simulink model "compare"  (R2018b)
settings: Solver=ode45  StartTime=0.0  StopTime=100  RelTol=1e-3
libraries: neural x79
(part 1 of 4)
settings Model: Creator=abinwa  LastModifiedBy=abinwa

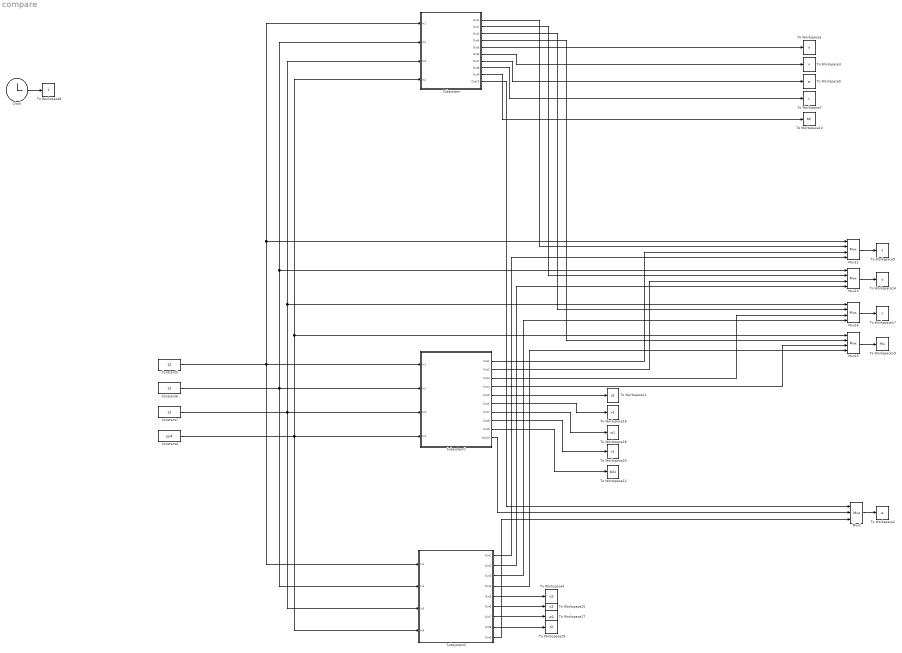
== system compare ==
  Clock : Clock
  Constant4 : Constant  Value=pi/4
  Constant5 : Constant  Value=12
  Constant6 : Constant  Value=12
  Constant7 : Constant  Value=12
  Mux1 : Mux  Inputs=3
  Mux{12..15} (4 alike) : Mux
  Subsystem : Subsystem
  Subsystem1 : Subsystem
  Subsystem2 : Subsystem
  To Workspace1 : ToWorkspace  VariableName=u  SampleTime=-1
  To Workspace10 : ToWorkspace  VariableName=tol  SampleTime=-1
  To Workspace11 : ToWorkspace  VariableName=u1  SampleTime=-1
  To Workspace12 : ToWorkspace  VariableName=tol1  SampleTime=-1
  To Workspace14 : ToWorkspace  VariableName=y  SampleTime=-1
  To Workspace16 : ToWorkspace  VariableName=v1  SampleTime=-1
  To Workspace17 : ToWorkspace  VariableName=z  SampleTime=-1
  To Workspace18 : ToWorkspace  VariableName=w1  SampleTime=-1
  To Workspace19 : ToWorkspace  VariableName=Psi  SampleTime=-1
  To Workspace2 : ToWorkspace  VariableName=e  SampleTime=-1
  To Workspace20 : ToWorkspace  VariableName=r1  SampleTime=-1
  To Workspace25 : ToWorkspace  VariableName=v2  SampleTime=-1
  To Workspace27 : ToWorkspace  VariableName=w2  SampleTime=-1
  To Workspace29 : ToWorkspace  VariableName=r2  SampleTime=-1
  To Workspace3 : ToWorkspace  VariableName=v  SampleTime=-1
  To Workspace4 : ToWorkspace  VariableName=u2  SampleTime=-1
  To Workspace5 : ToWorkspace  VariableName=w  SampleTime=-1
  To Workspace7 : ToWorkspace  VariableName=r  SampleTime=-1
  To Workspace8 : ToWorkspace  VariableName=t  SampleTime=-1
  To Workspace9 : ToWorkspace  VariableName=x  SampleTime=-1
  wires:
  Clock/1 -> To Workspace8/1
  Subsystem/1(Out1) -> Mux12/2
  Subsystem/2(Out2) -> Mux13/2
  Subsystem/3(Out3) -> Mux14/2
  Subsystem/4(Out4) -> Mux15/2
  Subsystem/5(Out5) -> To Workspace1/1
  Subsystem/6(Out6) -> To Workspace3/1
  Subsystem/7(Out7) -> To Workspace5/1
  Subsystem/8(Out8) -> To Workspace7/1
  Subsystem/9(Out9) -> To Workspace10/1
  Subsystem/10(Out10) -> Mux1/1
  Mux12/1 -> To Workspace9/1
  Mux13/1 -> To Workspace14/1
  Mux15/1 -> To Workspace19/1
  Constant5/1 -> Subsystem2/1(In1), Subsystem/1(In1), Mux12/1, Subsystem1/1(In1)
  Mux14/1 -> To Workspace17/1
  Constant6/1 -> Subsystem2/2(In2), Subsystem/2(In2), Mux13/1, Subsystem1/2(In2)
  Constant7/1 -> Subsystem2/3(In3), Subsystem1/3(In3), Subsystem/3(In3), Mux14/1
  Constant4/1 -> Subsystem2/4(In4), Subsystem1/4(In4), Subsystem/4(In4), Mux15/1
  Subsystem1/1(Out1) -> Mux12/3
  Subsystem1/2(Out2) -> Mux13/3
  Subsystem1/3(Out3) -> Mux14/3
  Subsystem1/4(Out4) -> Mux15/3
  Subsystem1/5(Out5) -> To Workspace11/1
  Subsystem1/6(Out6) -> To Workspace16/1
  Subsystem1/7(Out7) -> To Workspace18/1
  Subsystem1/8(Out8) -> To Workspace20/1
  Subsystem1/9(Out9) -> To Workspace12/1
  Subsystem1/10(Out10) -> Mux1/2
  Mux1/1 -> To Workspace2/1
  Subsystem2/1(Out1) -> Mux12/4
  Subsystem2/2(Out2) -> Mux13/4
  Subsystem2/3(Out3) -> Mux14/4
  Subsystem2/4(Out4) -> Mux15/4
  Subsystem2/5(Out5) -> To Workspace4/1
  Subsystem2/6(Out6) -> To Workspace25/1
  Subsystem2/7(Out7) -> To Workspace27/1
  Subsystem2/8(Out8) -> To Workspace29/1
  Subsystem2/9(Out9) -> Mux1/3

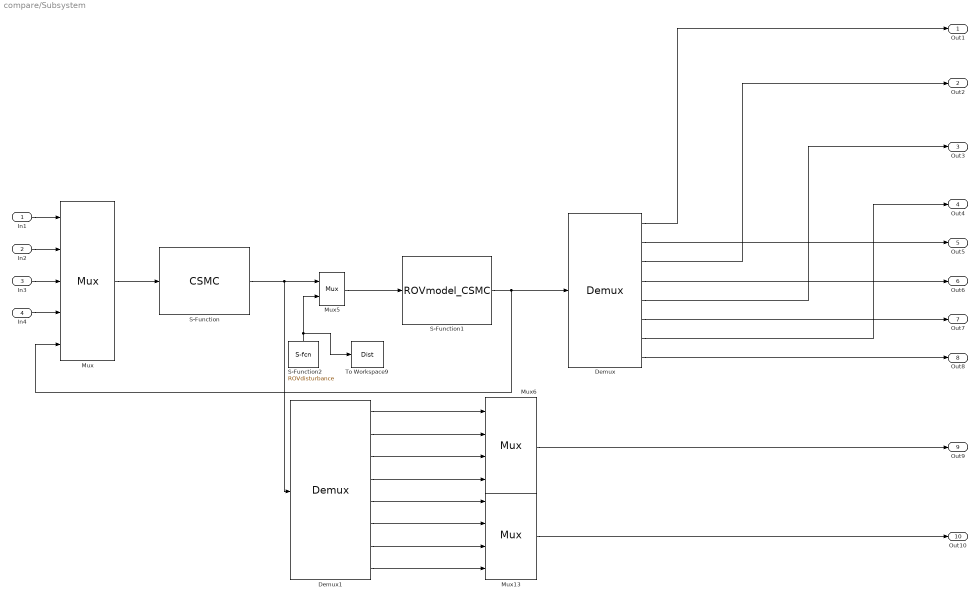
== system compare/Subsystem ==
  In1 : Inport
  In2 : Inport  Port=2
  In3 : Inport  Port=3
  In4 : Inport  Port=4
  Demux : Demux  Outputs=8
  Demux1 : Demux  Outputs=8
  Mux : Mux  Inputs=5
  Mux13 : Mux
  Mux5 : Mux  Inputs=2
  Mux6 : Mux
  S-Function : S-Function  FunctionName=CSMC  SFunctionDeploymentMode=off  EnableBusSupport=off
  S-Function1 : S-Function  FunctionName=ROVmodel_CSMC  SFunctionDeploymentMode=off  EnableBusSupport=off
  S-Function2 : S-Function  FunctionName=ROVdisturbance  SFunctionDeploymentMode=off  EnableBusSupport=off
  To Workspace9 : ToWorkspace  VariableName=Dist  SampleTime=-1
  Out1 : Outport
  Out2 : Outport  Port=2
  Out3 : Outport  Port=3
  Out4 : Outport  Port=4
  Out5 : Outport  Port=5
  Out6 : Outport  Port=6
  Out7 : Outport  Port=7
  Out8 : Outport  Port=8
  Out9 : Outport  Port=9
  Out10 : Outport  Port=10
  wires:
  Demux1/4 -> Mux6/4
  S-Function1/1 -> Demux/1, Mux/5
  Demux1/5 -> Mux13/1
  Demux/8 -> Out8/1
  Demux/5 -> Out3/1
  In3/1 -> Mux/3
  Demux1/1 -> Mux6/1
  Demux1/3 -> Mux6/3
  Demux1/2 -> Mux6/2
  Demux/7 -> Out4/1
  Mux5/1 -> S-Function1/1
  S-Function/1 -> Mux5/1, Demux1/1
  S-Function2/1 -> Mux5/2, To Workspace9/1
  Mux/1 -> S-Function/1
  Demux1/7 -> Mux13/3
  Demux1/6 -> Mux13/2
  Mux13/1 -> Out10/1
  Demux1/8 -> Mux13/4
  In1/1 -> Mux/1
  Demux/4 -> Out6/1
  In2/1 -> Mux/2
  Mux6/1 -> Out9/1
  Demux/3 -> Out2/1
  Demux/6 -> Out7/1
  Demux/2 -> Out5/1
  In4/1 -> Mux/4
  Demux/1 -> Out1/1

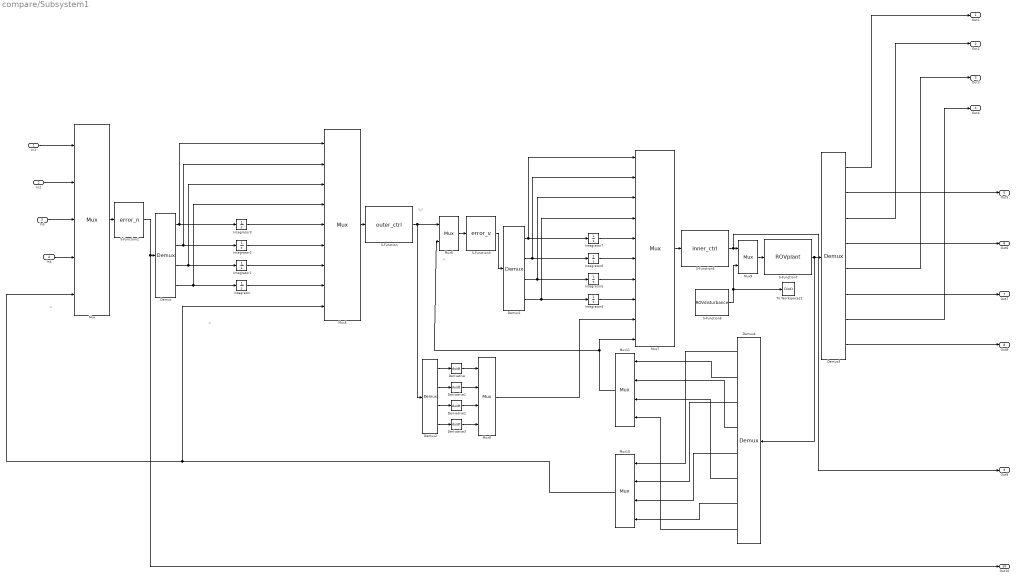
== system compare/Subsystem1 ==
  note: v_r
  note: n
  note: v
  note: n
  In1 : Inport
  In2 : Inport  Port=2
  In3 : Inport  Port=3
  In4 : Inport  Port=4
  Demux : Demux
  Demux1 : Demux
  Demux2 : Demux
  Demux3 : Demux  Outputs=8
  Demux4 : Demux  Outputs=8
  Derivative{,1..3} (4 alike) : Derivative
  Integrator{,1..7} (8 alike) : Integrator
  Mux : Mux  Inputs=5
  Mux10 : Mux
  Mux11 : Mux
  Mux5 : Mux  Inputs=9
  Mux6 : Mux  Inputs=2
  Mux7 : Mux  Inputs=10
  Mux8 : Mux
  Mux9 : Mux  Inputs=2
  S-Function : S-Function  FunctionName=outer_ctrl  SFunctionDeploymentMode=off  EnableBusSupport=off
  S-Function2 : S-Function  FunctionName=error_n  SFunctionDeploymentMode=off  EnableBusSupport=off
  S-Function3 : S-Function  FunctionName=error_v  SFunctionDeploymentMode=off  EnableBusSupport=off
  S-Function5 : S-Function  FunctionName=inner_ctrl  SFunctionDeploymentMode=off  EnableBusSupport=off
  S-Function6 : S-Function  FunctionName=ROVdisturbance  SFunctionDeploymentMode=off  EnableBusSupport=off
  S-Function7 : S-Function  FunctionName=ROVplant  SFunctionDeploymentMode=off  EnableBusSupport=off
  To Workspace21 : ToWorkspace  VariableName=Dist1  SampleTime=-1
  Out1 : Outport
  Out2 : Outport  Port=2
  Out3 : Outport  Port=3
  Out4 : Outport  Port=4
  Out5 : Outport  Port=5
  Out6 : Outport  Port=6
  Out7 : Outport  Port=7
  Out8 : Outport  Port=8
  Out9 : Outport  Port=9
  Out10 : Outport  Port=10
  wires:
  Demux1/4 -> Mux7/4, Integrator4/1
  S-Function6/1 -> To Workspace21/1, Mux9/2
  Mux8/1 -> Mux7/9
  Demux1/3 -> Mux7/3, Integrator5/1
  Demux2/2 -> Derivative1/1
  Demux4/5 -> Mux10/3
  Integrator/1 -> Mux5/8
  S-Function/1 -> Demux2/1, Mux6/1
  Integrator6/1 -> Mux7/6
  Integrator7/1 -> Mux7/5
  Mux9/1 -> S-Function7/1
  Mux10/1 -> Mux5/9, Mux/5
  Derivative3/1 -> Mux8/4
  Demux/1 -> Integrator3/1, Mux5/1
  Derivative2/1 -> Mux8/3
  S-Function3/1 -> Demux1/1
  S-Function7/1 -> Demux4/1, Demux3/1
  S-Function2/1 -> Out10/1, Demux/1
  Derivative/1 -> Mux8/1
  Demux4/2 -> Mux11/1
  Demux1/1 -> Mux7/1, Integrator7/1
  Mux11/1 -> Mux7/10, Mux6/2
  Mux5/1 -> S-Function/1
  Demux3/7 -> Out4/1
  Demux/4 -> Integrator/1, Mux5/4
  Demux2/3 -> Derivative2/1
  Integrator4/1 -> Mux7/8
  Mux/1 -> S-Function2/1
  Integrator2/1 -> Mux5/6
  Demux/2 -> Integrator2/1, Mux5/2
  Demux/3 -> Integrator1/1, Mux5/3
  Demux4/3 -> Mux10/2
  Derivative1/1 -> Mux8/2
  Mux6/1 -> S-Function3/1
  Demux3/1 -> Out1/1
  Mux7/1 -> S-Function5/1
  Integrator3/1 -> Mux5/5
  Demux4/4 -> Mux11/2
  Demux3/3 -> Out2/1
  Integrator1/1 -> Mux5/7
  Demux3/2 -> Out5/1
  Demux4/6 -> Mux11/3
  Integrator5/1 -> Mux7/7
  Demux4/8 -> Mux11/4
  Demux3/8 -> Out8/1
  Demux2/4 -> Derivative3/1
  Demux2/1 -> Derivative/1
  S-Function5/1 -> Out9/1, Mux9/1
  Demux1/2 -> Mux7/2, Integrator6/1
  Demux4/7 -> Mux10/4
  Demux4/1 -> Mux10/1
  In3/1 -> Mux/3
  Demux3/4 -> Out6/1
  In4/1 -> Mux/4
  Demux3/5 -> Out3/1
  Demux3/6 -> Out7/1
  In2/1 -> Mux/2
  In1/1 -> Mux/1

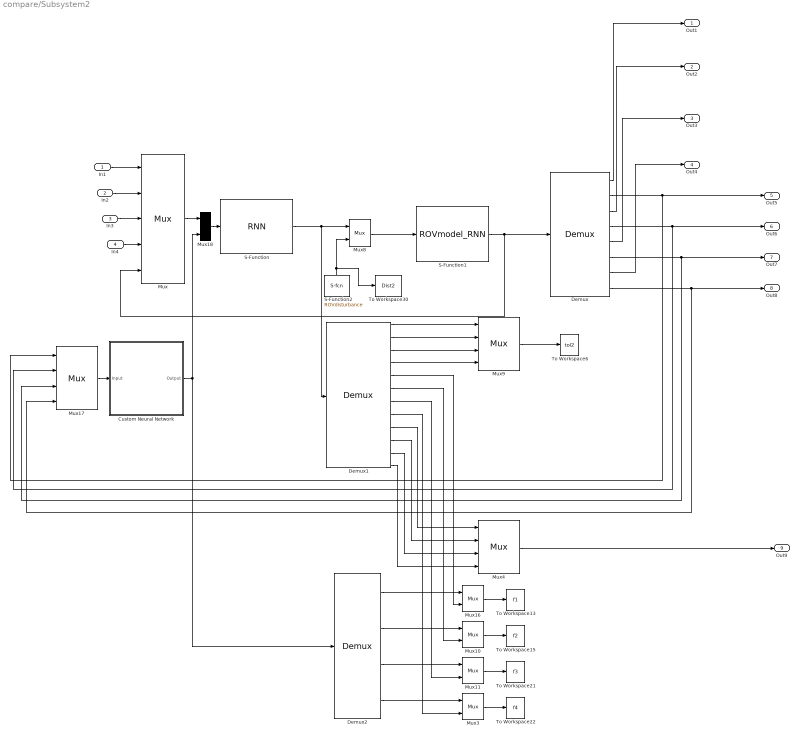
== system compare/Subsystem2 ==
  In1 : Inport
  In2 : Inport  Port=2
  In3 : Inport  Port=3
  In4 : Inport  Port=4
  Custom Neural Network : Subsystem  mask{ai_layer_1_delayed_1=[0;0;0;0;0;0;0;0;0;0;0;0;0;0;0;0;0;0;0;0], ai_layer_2_delayed_1=[0;0;0;0;0;0;0;0;0;0;0;0;0;0;0]}
      mask prompts: ai_layer_1_delayed_1 "Initial layer 1 state at timestep 0."; ai_layer_2_delayed_1 "Initial layer 2 state at timestep 0."
      mask help: Custom Neural Network
      mask Display: e = 0.06;c1 = [120 150 230]/255;c2 = ([120 150 230]+0)/383;c3 = ([120 150 230]+128)/383;patch([0 1 1 0],[0 0 1 1],c1);patch([0 1 1 1-e 1-e 0+e],[0 0 1 1-e 0+e 0+e],c2);patch([0 0 1 1-e 0+e 0+e],[0 1 1 1-e 1-e 0+e],c3);plot([0 1 1 0 0],[0 0 1 1 0]);fprintf('NNET');port_label('input',1,' Input');port_label('output',1,'Output ');
  Demux : Demux  Outputs=8
  Demux1 : Demux  Outputs=12
  Demux2 : Demux
  Mux : Mux  Inputs=5
  Mux{3,8,10..11,16,18} (6 alike) : Mux  Inputs=2
  Mux17 : Mux
  Mux4 : Mux
  Mux9 : Mux
  S-Function : S-Function  FunctionName=RNN  SFunctionDeploymentMode=off  EnableBusSupport=off
  S-Function1 : S-Function  FunctionName=ROVmodel_RNN  SFunctionDeploymentMode=off  EnableBusSupport=off
  S-Function2 : S-Function  FunctionName=ROVdisturbance  SFunctionDeploymentMode=off  EnableBusSupport=off
  To Workspace13 : ToWorkspace  VariableName=f1  SampleTime=-1
  To Workspace15 : ToWorkspace  VariableName=f2  SampleTime=-1
  To Workspace21 : ToWorkspace  VariableName=f3  SampleTime=-1
  To Workspace22 : ToWorkspace  VariableName=f4  SampleTime=-1
  To Workspace30 : ToWorkspace  VariableName=Dist2  SampleTime=-1
  To Workspace6 : ToWorkspace  VariableName=tol2  SampleTime=-1
  Out1 : Outport
  Out2 : Outport  Port=2
  Out3 : Outport  Port=3
  Out4 : Outport  Port=4
  Out5 : Outport  Port=5
  Out6 : Outport  Port=6
  Out7 : Outport  Port=7
  Out8 : Outport  Port=8
  Out9 : Outport  Port=9
  wires:
  Demux2/3 -> Mux11/1
  S-Function1/1 -> Demux/1, Mux/5
  Demux/4 -> Out6/1, Mux17/2
  Demux/2 -> Out5/1, Mux17/1
  Demux1/10 -> Mux4/2
  Demux2/2 -> Mux10/1
  Mux11/1 -> To Workspace21/1
  Demux1/6 -> Mux10/2
  In3/1 -> Mux/3
  In1/1 -> Mux/1
  Demux1/1 -> Mux9/1
  Demux/6 -> Out7/1, Mux17/3
  Demux1/4 -> Mux9/4
  Demux1/12 -> Mux4/4
  Mux9/1 -> To Workspace6/1
  Demux1/2 -> Mux9/2
  Mux18/1 -> S-Function/1
  Mux8/1 -> S-Function1/1
  Mux17/1 -> Custom Neural Network/1(Input)
  Demux1/5 -> Mux16/2
  S-Function/1 -> Mux8/1, Demux1/1
  Custom Neural Network/1(Output) -> Mux18/2, Demux2/1
  Demux/3 -> Out2/1
  Demux2/4 -> Mux3/1
  Mux3/1 -> To Workspace22/1
  Mux16/1 -> To Workspace13/1
  Demux/5 -> Out3/1
  Demux1/9 -> Mux4/1
  In2/1 -> Mux/2
  Demux1/11 -> Mux4/3
  Demux/8 -> Out8/1, Mux17/4
  Demux1/8 -> Mux3/2
  Mux/1 -> Mux18/1
  S-Function2/1 -> Mux8/2, To Workspace30/1
  Demux1/7 -> Mux11/2
  Demux2/1 -> Mux16/1
  Mux10/1 -> To Workspace15/1
  Demux1/3 -> Mux9/3
  Demux/7 -> Out4/1
  In4/1 -> Mux/4
  Demux/1 -> Out1/1
  Mux4/1 -> Out9/1

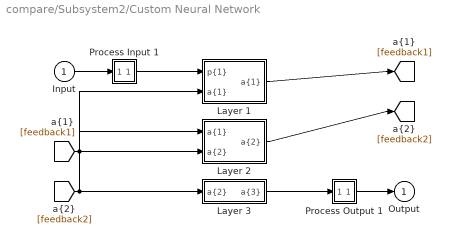
== system compare/Subsystem2/Custom Neural Network ==
  Input : Inport  PortDimensions=4  SampleTime=1
      mask Display: e = 0.06;c1 = [120 230 180]/255;c2 = ([120 230 180]+0)/(256+128);c3 = ([120 230 180]+128)/(256+128);patch([0 1 1 0],[0 0 1 1],c1);patch([0 1 1 1-e 1-e 0+e],[0 0 1 1-e 0+e 0+e],c2);patch([0 0 1 1-e 0+e 0+e],[0 1 1 1-e 1-e 0+e],c3);plot([0 1 1 0 0],[0 0 1 1 0]);
  Layer 1 : Subsystem
      mask Display: e = 0.06;c1 = [120 150 230]/255;c2 = ([120 150 230]+0)/383;c3 = ([120 150 230]+128)/383;patch([0 1 1 0],[0 0 1 1],c1);patch([0 1 1 1-e 1-e 0+e],[0 0 1 1-e 0+e 0+e],c2);patch([0 0 1 1-e 0+e 0+e],[0 1 1 1-e 1-e 0+e],c3);plot([0 1 1 0 0],[0 0 1 1 0]);
  Layer 2 : Subsystem
      mask Display: e = 0.06;c1 = [120 150 230]/255;c2 = ([120 150 230]+0)/383;c3 = ([120 150 230]+128)/383;patch([0 1 1 0],[0 0 1 1],c1);patch([0 1 1 1-e 1-e 0+e],[0 0 1 1-e 0+e 0+e],c2);patch([0 0 1 1-e 0+e 0+e],[0 1 1 1-e 1-e 0+e],c3);plot([0 1 1 0 0],[0 0 1 1 0]);
  Layer 3 : Subsystem
      mask Display: e = 0.06;c1 = [120 150 230]/255;c2 = ([120 150 230]+0)/383;c3 = ([120 150 230]+128)/383;patch([0 1 1 0],[0 0 1 1],c1);patch([0 1 1 1-e 1-e 0+e],[0 0 1 1-e 0+e 0+e],c2);patch([0 0 1 1-e 0+e 0+e],[0 1 1 1-e 1-e 0+e],c3);plot([0 1 1 0 0],[0 0 1 1 0]);
  Process Input 1 : Subsystem
      mask Display: e = 0.06;c1 = [120 150 230]/255;c2 = ([120 150 230]+0)/383;c3 = ([120 150 230]+128)/383;patch([0 1 1 0],[0 0 1 1],c1);patch([0 1 1 1-e 1-e 0+e],[0 0 1 1-e 0+e 0+e],c2);patch([0 0 1 1-e 0+e 0+e],[0 1 1 1-e 1-e 0+e],c3);plot([0 1 1 0 0],[0 0 1 1 0]);
  Process Output 1 : Subsystem
      mask Display: e = 0.06;c1 = [120 150 230]/255;c2 = ([120 150 230]+0)/383;c3 = ([120 150 230]+128)/383;patch([0 1 1 0],[0 0 1 1],c1);patch([0 1 1 1-e 1-e 0+e],[0 0 1 1-e 0+e 0+e],c2);patch([0 0 1 1-e 0+e 0+e],[0 1 1 1-e 1-e 0+e],c3);plot([0 1 1 0 0],[0 0 1 1 0]);
  Output : Outport  InitialOutput=[0;0;0;0]
      mask Display: e = 0.06;c1 = [120 230 180]/255;c2 = ([120 230 180]+0)/(256+128);c3 = ([120 230 180]+128)/(256+128);patch([0 1 1 0],[0 0 1 1],c1);patch([0 1 1 1-e 1-e 0+e],[0 0 1 1-e 0+e 0+e],c2);patch([0 0 1 1-e 0+e 0+e],[0 1 1 1-e 1-e 0+e],c3);plot([0 1 1 0 0],[0 0 1 1 0]);
  wires:
  Input/1 -> Process Input 1/1(x)
  Process Output 1/1(y) -> Output/1
  Process Input 1/1(p) -> Layer 1/1("p{1}")
  Layer 1/1("a{1}") -> [feedback1]
  [feedback1] -> Layer 1/2("a{1} "), Layer 2/1("a{1} ")
  Layer 2/1("a{2}") -> [feedback2]
  [feedback2] -> Layer 2/2("a{2} "), Layer 3/1("a{2} ")
  Layer 3/1("a{3}") -> Process Output 1/1(a)

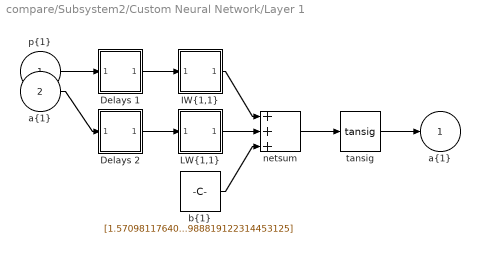
== system compare/Subsystem2/Custom Neural Network/Layer 1 ==
  "p{1}" : Inport  PortDimensions=4  SampleTime=1
      mask Display: e = 0.06;c1 = [120 230 180]/255;c2 = ([120 230 180]+0)/(256+128);c3 = ([120 230 180]+128)/(256+128);patch([0 1 1 0],[0 0 1 1],c1);patch([0 1 1 1-e 1-e 0+e],[0 0 1 1-e 0+e 0+e],c2);patch([0 0 1 1-e 0+e 0+e],[0 1 1 1-e 1-e 0+e],c3);plot([0 1 1 0 0],[0 0 1 1 0]);
  "a{1} " : Inport  Port=2  PortDimensions=20  SampleTime=1
      mask Display: e = 0.06;c1 = [120 230 180]/255;c2 = ([120 230 180]+0)/(256+128);c3 = ([120 230 180]+128)/(256+128);patch([0 1 1 0],[0 0 1 1],c1);patch([0 1 1 1-e 1-e 0+e],[0 0 1 1-e 0+e 0+e],c2);patch([0 0 1 1-e 0+e 0+e],[0 1 1 1-e 1-e 0+e],c3);plot([0 1 1 0 0],[0 0 1 1 0]);
  Delays 1 : Subsystem
      mask Display: e = 0.06;c1 = [120 150 230]/255;c2 = ([120 150 230]+0)/383;c3 = ([120 150 230]+128)/383;patch([0 1 1 0],[0 0 1 1],c1);patch([0 1 1 1-e 1-e 0+e],[0 0 1 1-e 0+e 0+e],c2);patch([0 0 1 1-e 0+e 0+e],[0 1 1 1-e 1-e 0+e],c3);plot([0 1 1 0 0],[0 0 1 1 0]);disp('0');
  Delays 2 : Subsystem
      mask Display: e = 0.06;c1 = [120 150 230]/255;c2 = ([120 150 230]+0)/383;c3 = ([120 150 230]+128)/383;patch([0 1 1 0],[0 0 1 1],c1);patch([0 1 1 1-e 1-e 0+e],[0 0 1 1-e 0+e 0+e],c2);patch([0 0 1 1-e 0+e 0+e],[0 1 1 1-e 1-e 0+e],c3);plot([0 1 1 0 0],[0 0 1 1 0]);disp('1');
  "IW{1,1}" : Subsystem
      mask Display: e = 0.06;c1 = [120 150 230]/255;c2 = ([120 150 230]+0)/383;c3 = ([120 150 230]+128)/383;patch([0 1 1 0],[0 0 1 1],c1);patch([0 1 1 1-e 1-e 0+e],[0 0 1 1-e 0+e 0+e],c2);patch([0 0 1 1-e 0+e 0+e],[0 1 1 1-e 1-e 0+e],c3);plot([0 1 1 0 0],[0 0 1 1 0]);disp('W');
  "LW{1,1}" : Subsystem
      mask Display: e = 0.06;c1 = [120 150 230]/255;c2 = ([120 150 230]+0)/383;c3 = ([120 150 230]+128)/383;patch([0 1 1 0],[0 0 1 1],c1);patch([0 1 1 1-e 1-e 0+e],[0 0 1 1-e 0+e 0+e],c2);patch([0 0 1 1-e 0+e 0+e],[0 1 1 1-e 1-e 0+e],c3);plot([0 1 1 0 0],[0 0 1 1 0]);disp('W');
  "b{1}" : Constant  Value=[1.5709811764087333596506823596428148448467254638671875;-1.422432849296332957322874790406785905361175537109375;1.257830636243737476576143308193422853946685791015625;-1.0965606272778114504973245857399888336658477783203125;-0.93559678076312768890687721068388782441616058349609375;-0.73655566333232591613722206602687947452068328857421875;-0.50859059257384853225403276155702769756317138671875;-0.3661309918072708224912048535770736634731292724609375;0.2362124825473512768070349920890294015407562255859375;0.0871527292053556890127907763599068857729434967041015625;-0.09220173179144837416476576663626474328339099884033203125;0.201297008489096651562277884295326657593250274658203125;0.40818274931037457076143937229062430560588836669921875;-0.612669858552886470448584077530540525913238525390625;0.79439985267361856724477320312871597707271575927734375;0.8775296810612600584278197857202030718326568603515625;1.0930187382606926238537425888353027403354644775390625;1.2798307915173892101989849834353663027286529541015625;-1.3805805253881249239356066027539782226085662841796875;-1.5889086928901339224040611952659673988819122314453125]
      mask Display: e = 0.06;c1 = [120 150 230]/255;c2 = ([120 150 230]+0)/383;c3 = ([120 150 230]+128)/383;patch([0 1 1 0],[0 0 1 1],c1);patch([0 1 1 1-e 1-e 0+e],[0 0 1 1-e 0+e 0+e],c2);patch([0 0 1 1-e 0+e 0+e],[0 1 1 1-e 1-e 0+e],c3);plot([0 1 1 0 0],[0 0 1 1 0]);disp('b');
  netsum : Sum  Inputs=3  SaturateOnIntegerOverflow=on  InputSameDT=on  OutDataTypeStr=Inherit: Same as first input
      mask Display: e = 0.06;c1 = [120 150 230]/255;c2 = ([120 150 230]+0)/383;c3 = ([120 150 230]+128)/383;patch([0 1 1 0],[0 0 1 1],c1);patch([0 1 1 1-e 1-e 0+e],[0 0 1 1-e 0+e 0+e],c2);patch([0 0 1 1-e 0+e 0+e],[0 1 1 1-e 1-e 0+e],c3);plot([0 1 1 0 0],[0 0 1 1 0]);disp('+');
  tansig : neural/Transfer Functions/tansig
  "a{1}" : Outport  InitialOutput=[0;0;0;0;0;0;0;0;0;0;0;0;0;0;0;0;0;0;0;0]
      mask Display: e = 0.06;c1 = [120 230 180]/255;c2 = ([120 230 180]+0)/(256+128);c3 = ([120 230 180]+128)/(256+128);patch([0 1 1 0],[0 0 1 1],c1);patch([0 1 1 1-e 1-e 0+e],[0 0 1 1-e 0+e 0+e],c2);patch([0 0 1 1-e 0+e 0+e],[0 1 1 1-e 1-e 0+e],c3);plot([0 1 1 0 0],[0 0 1 1 0]);
  wires:
  "p{1}"/1 -> Delays 1/1("p{1}")
  Delays 1/1("pd{1,1}") -> "IW{1,1}"/1("pd{1,1}")
  "IW{1,1}"/1("iz{1,1}") -> netsum/1
  "a{1} "/1 -> Delays 2/1("p{1}")
  Delays 2/1("pd{1,1}") -> "LW{1,1}"/1("ad{1,1}")
  "LW{1,1}"/1("lz{1,1}") -> netsum/2
  "b{1}"/1 -> netsum/3
  netsum/1 -> tansig/1
  tansig/1 -> "a{1}"/1

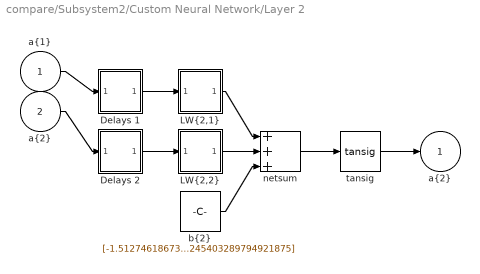
== system compare/Subsystem2/Custom Neural Network/Layer 2 ==
  "a{1} " : Inport  PortDimensions=20  SampleTime=1
      mask Display: e = 0.06;c1 = [120 230 180]/255;c2 = ([120 230 180]+0)/(256+128);c3 = ([120 230 180]+128)/(256+128);patch([0 1 1 0],[0 0 1 1],c1);patch([0 1 1 1-e 1-e 0+e],[0 0 1 1-e 0+e 0+e],c2);patch([0 0 1 1-e 0+e 0+e],[0 1 1 1-e 1-e 0+e],c3);plot([0 1 1 0 0],[0 0 1 1 0]);
  "a{2} " : Inport  Port=2  PortDimensions=15  SampleTime=1
      mask Display: e = 0.06;c1 = [120 230 180]/255;c2 = ([120 230 180]+0)/(256+128);c3 = ([120 230 180]+128)/(256+128);patch([0 1 1 0],[0 0 1 1],c1);patch([0 1 1 1-e 1-e 0+e],[0 0 1 1-e 0+e 0+e],c2);patch([0 0 1 1-e 0+e 0+e],[0 1 1 1-e 1-e 0+e],c3);plot([0 1 1 0 0],[0 0 1 1 0]);
  Delays 1 : Subsystem
      mask Display: e = 0.06;c1 = [120 150 230]/255;c2 = ([120 150 230]+0)/383;c3 = ([120 150 230]+128)/383;patch([0 1 1 0],[0 0 1 1],c1);patch([0 1 1 1-e 1-e 0+e],[0 0 1 1-e 0+e 0+e],c2);patch([0 0 1 1-e 0+e 0+e],[0 1 1 1-e 1-e 0+e],c3);plot([0 1 1 0 0],[0 0 1 1 0]);disp('0');
  Delays 2 : Subsystem
      mask Display: e = 0.06;c1 = [120 150 230]/255;c2 = ([120 150 230]+0)/383;c3 = ([120 150 230]+128)/383;patch([0 1 1 0],[0 0 1 1],c1);patch([0 1 1 1-e 1-e 0+e],[0 0 1 1-e 0+e 0+e],c2);patch([0 0 1 1-e 0+e 0+e],[0 1 1 1-e 1-e 0+e],c3);plot([0 1 1 0 0],[0 0 1 1 0]);disp('1');
  "LW{2,1}" : Subsystem
      mask Display: e = 0.06;c1 = [120 150 230]/255;c2 = ([120 150 230]+0)/383;c3 = ([120 150 230]+128)/383;patch([0 1 1 0],[0 0 1 1],c1);patch([0 1 1 1-e 1-e 0+e],[0 0 1 1-e 0+e 0+e],c2);patch([0 0 1 1-e 0+e 0+e],[0 1 1 1-e 1-e 0+e],c3);plot([0 1 1 0 0],[0 0 1 1 0]);disp('W');
  "LW{2,2}" : Subsystem
      mask Display: e = 0.06;c1 = [120 150 230]/255;c2 = ([120 150 230]+0)/383;c3 = ([120 150 230]+128)/383;patch([0 1 1 0],[0 0 1 1],c1);patch([0 1 1 1-e 1-e 0+e],[0 0 1 1-e 0+e 0+e],c2);patch([0 0 1 1-e 0+e 0+e],[0 1 1 1-e 1-e 0+e],c3);plot([0 1 1 0 0],[0 0 1 1 0]);disp('W');
  "b{2}" : Constant  Value=[-1.5127461867306031262359056199784390628337860107421875;-1.3120033471746694875292860160698182880878448486328125;1.074781860594610893855360700399614870548248291015625;-0.83144301510085683037942771989037282764911651611328125;-0.69278289828230532609865122140035964548587799072265625;-0.40771218671634346097931711483397521078586578369140625;0.220712656388276418084615215775556862354278564453125;0.015832253557886068195958984006210812367498874664306640625;-0.1745475244332462538832118070786236785352230072021484375;0.428927670355808976498934725896106101572513580322265625;-0.72270774537646798041379270216566510498523712158203125;0.835492180685874163970083827734924852848052978515625;-1.05916229113629700719911852502264082431793212890625;-1.291611524553415879523754483670927584171295166015625;1.445844010598943185641473974101245403289794921875]
      mask Display: e = 0.06;c1 = [120 150 230]/255;c2 = ([120 150 230]+0)/383;c3 = ([120 150 230]+128)/383;patch([0 1 1 0],[0 0 1 1],c1);patch([0 1 1 1-e 1-e 0+e],[0 0 1 1-e 0+e 0+e],c2);patch([0 0 1 1-e 0+e 0+e],[0 1 1 1-e 1-e 0+e],c3);plot([0 1 1 0 0],[0 0 1 1 0]);disp('b');
  netsum : Sum  Inputs=3  SaturateOnIntegerOverflow=on  InputSameDT=on  OutDataTypeStr=Inherit: Same as first input
      mask Display: e = 0.06;c1 = [120 150 230]/255;c2 = ([120 150 230]+0)/383;c3 = ([120 150 230]+128)/383;patch([0 1 1 0],[0 0 1 1],c1);patch([0 1 1 1-e 1-e 0+e],[0 0 1 1-e 0+e 0+e],c2);patch([0 0 1 1-e 0+e 0+e],[0 1 1 1-e 1-e 0+e],c3);plot([0 1 1 0 0],[0 0 1 1 0]);disp('+');
  tansig : neural/Transfer Functions/tansig
  "a{2}" : Outport  InitialOutput=[0;0;0;0;0;0;0;0;0;0;0;0;0;0;0]
      mask Display: e = 0.06;c1 = [120 230 180]/255;c2 = ([120 230 180]+0)/(256+128);c3 = ([120 230 180]+128)/(256+128);patch([0 1 1 0],[0 0 1 1],c1);patch([0 1 1 1-e 1-e 0+e],[0 0 1 1-e 0+e 0+e],c2);patch([0 0 1 1-e 0+e 0+e],[0 1 1 1-e 1-e 0+e],c3);plot([0 1 1 0 0],[0 0 1 1 0]);
  wires:
  "a{1} "/1 -> Delays 1/1("p{2}")
  Delays 1/1("pd{2,1}") -> "LW{2,1}"/1("ad{2,1}")
  "LW{2,1}"/1("lz{2,1}") -> netsum/1
  "a{2} "/1 -> Delays 2/1("p{2}")
  Delays 2/1("pd{2,2}") -> "LW{2,2}"/1("ad{2,2}")
  "LW{2,2}"/1("lz{2,2}") -> netsum/2
  "b{2}"/1 -> netsum/3
  netsum/1 -> tansig/1
  tansig/1 -> "a{2}"/1

== system compare/Subsystem2/Custom Neural Network/Layer 3 ==
  "a{2} " : Inport  PortDimensions=15  SampleTime=1
      mask Display: e = 0.06;c1 = [120 230 180]/255;c2 = ([120 230 180]+0)/(256+128);c3 = ([120 230 180]+128)/(256+128);patch([0 1 1 0],[0 0 1 1],c1);patch([0 1 1 1-e 1-e 0+e],[0 0 1 1-e 0+e 0+e],c2);patch([0 0 1 1-e 0+e 0+e],[0 1 1 1-e 1-e 0+e],c3);plot([0 1 1 0 0],[0 0 1 1 0]);
  Delays 1 : Subsystem
      mask Display: e = 0.06;c1 = [120 150 230]/255;c2 = ([120 150 230]+0)/383;c3 = ([120 150 230]+128)/383;patch([0 1 1 0],[0 0 1 1],c1);patch([0 1 1 1-e 1-e 0+e],[0 0 1 1-e 0+e 0+e],c2);patch([0 0 1 1-e 0+e 0+e],[0 1 1 1-e 1-e 0+e],c3);plot([0 1 1 0 0],[0 0 1 1 0]);disp('0');
  "LW{3,2}" : Subsystem
      mask Display: e = 0.06;c1 = [120 150 230]/255;c2 = ([120 150 230]+0)/383;c3 = ([120 150 230]+128)/383;patch([0 1 1 0],[0 0 1 1],c1);patch([0 1 1 1-e 1-e 0+e],[0 0 1 1-e 0+e 0+e],c2);patch([0 0 1 1-e 0+e 0+e],[0 1 1 1-e 1-e 0+e],c3);plot([0 1 1 0 0],[0 0 1 1 0]);disp('W');
  "b{3}" : Constant  Value=[-1.6513168917505269828183145364164374768733978271484375;-0.53390046225428733350781840272247791290283203125;-0.511851706610572332323272348730824887752532958984375;-1.513230267073728985138814095989800989627838134765625]
      mask Display: e = 0.06;c1 = [120 150 230]/255;c2 = ([120 150 230]+0)/383;c3 = ([120 150 230]+128)/383;patch([0 1 1 0],[0 0 1 1],c1);patch([0 1 1 1-e 1-e 0+e],[0 0 1 1-e 0+e 0+e],c2);patch([0 0 1 1-e 0+e 0+e],[0 1 1 1-e 1-e 0+e],c3);plot([0 1 1 0 0],[0 0 1 1 0]);disp('b');
  netsum : Sum  Inputs=2  SaturateOnIntegerOverflow=on  InputSameDT=on  OutDataTypeStr=Inherit: Same as first input
      mask Display: e = 0.06;c1 = [120 150 230]/255;c2 = ([120 150 230]+0)/383;c3 = ([120 150 230]+128)/383;patch([0 1 1 0],[0 0 1 1],c1);patch([0 1 1 1-e 1-e 0+e],[0 0 1 1-e 0+e 0+e],c2);patch([0 0 1 1-e 0+e 0+e],[0 1 1 1-e 1-e 0+e],c3);plot([0 1 1 0 0],[0 0 1 1 0]);disp('+');
  tansig : neural/Transfer Functions/tansig
  "a{3}" : Outport  InitialOutput=[0;0;0;0]
      mask Display: e = 0.06;c1 = [120 230 180]/255;c2 = ([120 230 180]+0)/(256+128);c3 = ([120 230 180]+128)/(256+128);patch([0 1 1 0],[0 0 1 1],c1);patch([0 1 1 1-e 1-e 0+e],[0 0 1 1-e 0+e 0+e],c2);patch([0 0 1 1-e 0+e 0+e],[0 1 1 1-e 1-e 0+e],c3);plot([0 1 1 0 0],[0 0 1 1 0]);
  wires:
  "a{2} "/1 -> Delays 1/1("p{3}")
  Delays 1/1("pd{3,2}") -> "LW{3,2}"/1("ad{3,2}")
  "LW{3,2}"/1("lz{3,2}") -> netsum/1
  "b{3}"/1 -> netsum/2
  netsum/1 -> tansig/1
  tansig/1 -> "a{3}"/1

== system compare/Subsystem2/Custom Neural Network/Process Input 1 ==
  x : Inport  PortDimensions=4  SampleTime=1
      mask Display: e = 0.06;c1 = [120 230 180]/255;c2 = ([120 230 180]+0)/(256+128);c3 = ([120 230 180]+128)/(256+128);patch([0 1 1 0],[0 0 1 1],c1);patch([0 1 1 1-e 1-e 0+e],[0 0 1 1-e 0+e 0+e],c2);patch([0 0 1 1-e 0+e 0+e],[0 1 1 1-e 1-e 0+e],c3);plot([0 1 1 0 0],[0 0 1 1 0]);
  mapminmax : neural/Processing Functions/mapminmax  xmin=[-1.00404523544620993824594279431;-1.00860631769114994504832338862;0;-13.8476689246916002673515322385]  xmax=[95.6496884063110996976320166141;229.551115094576999808850814588;1.15180418978859000489478603413;0.0162883524021428006955947154211]  ymin=-1  ymax=1
  p : Outport  PortDimensions=4  SampleTime=1
      mask Display: e = 0.06;c1 = [120 230 180]/255;c2 = ([120 230 180]+0)/(256+128);c3 = ([120 230 180]+128)/(256+128);patch([0 1 1 0],[0 0 1 1],c1);patch([0 1 1 1-e 1-e 0+e],[0 0 1 1-e 0+e 0+e],c2);patch([0 0 1 1-e 0+e 0+e],[0 1 1 1-e 1-e 0+e],c3);plot([0 1 1 0 0],[0 0 1 1 0]);
  wires:
  x/1 -> mapminmax/1
  mapminmax/1 -> p/1

== system compare/Subsystem2/Custom Neural Network/Process Output 1 ==
  a : Inport  PortDimensions=4  SampleTime=1
      mask Display: e = 0.06;c1 = [120 230 180]/255;c2 = ([120 230 180]+0)/(256+128);c3 = ([120 230 180]+128)/(256+128);patch([0 1 1 0],[0 0 1 1],c1);patch([0 1 1 1-e 1-e 0+e],[0 0 1 1-e 0+e 0+e],c2);patch([0 0 1 1-e 0+e 0+e],[0 1 1 1-e 1-e 0+e],c3);plot([0 1 1 0 0],[0 0 1 1 0]);
  mapminmax_reverse : neural/Processing Functions/mapminmax_reverse  xmin=[-14.0342489334772952958019232028;-9.64963841204492744907383894315;-0.160000000000000003330669073875;0]  xmax=[58682.0588991207187063992023468;131842.055516550084576010704041;8.68480066186182142473626299761;672976.876018791226670145988464]  ymin=-1  ymax=1
  y : Outport  PortDimensions=4  SampleTime=1
      mask Display: e = 0.06;c1 = [120 230 180]/255;c2 = ([120 230 180]+0)/(256+128);c3 = ([120 230 180]+128)/(256+128);patch([0 1 1 0],[0 0 1 1],c1);patch([0 1 1 1-e 1-e 0+e],[0 0 1 1-e 0+e 0+e],c2);patch([0 0 1 1-e 0+e 0+e],[0 1 1 1-e 1-e 0+e],c3);plot([0 1 1 0 0],[0 0 1 1 0]);
  wires:
  a/1 -> mapminmax_reverse/1
  mapminmax_reverse/1 -> y/1

== system compare/Subsystem2/Custom Neural Network/Layer 1/Delays 1 ==
  "p{1}" : Inport  PortDimensions=4  SampleTime=1
      mask Display: e = 0.06;c1 = [120 230 180]/255;c2 = ([120 230 180]+0)/(256+128);c3 = ([120 230 180]+128)/(256+128);patch([0 1 1 0],[0 0 1 1],c1);patch([0 1 1 1-e 1-e 0+e],[0 0 1 1-e 0+e 0+e],c2);patch([0 0 1 1-e 0+e 0+e],[0 1 1 1-e 1-e 0+e],c3);plot([0 1 1 0 0],[0 0 1 1 0]);
  mux : Mux  Inputs=1
      mask Display: e = 0.06;c1 = [120 150 230]/255;c2 = ([120 150 230]+0)/383;c3 = ([120 150 230]+128)/383;patch([0 1 1 0],[0 0 1 1],c1);patch([0 1 1 1-e 1-e 0+e],[0 0 1 1-e 0+e 0+e],c2);patch([0 0 1 1-e 0+e 0+e],[0 1 1 1-e 1-e 0+e],c3);plot([0 1 1 0 0],[0 0 1 1 0]);disp('Mux')
  "pd{1,1}" : Outport
      mask Display: e = 0.06;c1 = [120 230 180]/255;c2 = ([120 230 180]+0)/(256+128);c3 = ([120 230 180]+128)/(256+128);patch([0 1 1 0],[0 0 1 1],c1);patch([0 1 1 1-e 1-e 0+e],[0 0 1 1-e 0+e 0+e],c2);patch([0 0 1 1-e 0+e 0+e],[0 1 1 1-e 1-e 0+e],c3);plot([0 1 1 0 0],[0 0 1 1 0]);
  wires:
  "p{1}"/1 -> mux/1
  mux/1 -> "pd{1,1}"/1

== system compare/Subsystem2/Custom Neural Network/Layer 1/Delays 2 ==
  "p{1}" : Inport  PortDimensions=20  SampleTime=1
      mask Display: e = 0.06;c1 = [120 230 180]/255;c2 = ([120 230 180]+0)/(256+128);c3 = ([120 230 180]+128)/(256+128);patch([0 1 1 0],[0 0 1 1],c1);patch([0 1 1 1-e 1-e 0+e],[0 0 1 1-e 0+e 0+e],c2);patch([0 0 1 1-e 0+e 0+e],[0 1 1 1-e 1-e 0+e],c3);plot([0 1 1 0 0],[0 0 1 1 0]);
  Delay 1 : UnitDelay  InitialCondition=ai_layer_1_delayed_1
      mask Display: e = 0.06;c1 = [120 150 230]/255;c2 = ([120 150 230]+0)/383;c3 = ([120 150 230]+128)/383;patch([0 1 1 0],[0 0 1 1],c1);patch([0 1 1 1-e 1-e 0+e],[0 0 1 1-e 0+e 0+e],c2);patch([0 0 1 1-e 0+e 0+e],[0 1 1 1-e 1-e 0+e],c3);plot([0 1 1 0 0],[0 0 1 1 0]);disp('D')
  mux : Mux  Inputs=1
      mask Display: e = 0.06;c1 = [120 150 230]/255;c2 = ([120 150 230]+0)/383;c3 = ([120 150 230]+128)/383;patch([0 1 1 0],[0 0 1 1],c1);patch([0 1 1 1-e 1-e 0+e],[0 0 1 1-e 0+e 0+e],c2);patch([0 0 1 1-e 0+e 0+e],[0 1 1 1-e 1-e 0+e],c3);plot([0 1 1 0 0],[0 0 1 1 0]);disp('Mux')
  "pd{1,1}" : Outport
      mask Display: e = 0.06;c1 = [120 230 180]/255;c2 = ([120 230 180]+0)/(256+128);c3 = ([120 230 180]+128)/(256+128);patch([0 1 1 0],[0 0 1 1],c1);patch([0 1 1 1-e 1-e 0+e],[0 0 1 1-e 0+e 0+e],c2);patch([0 0 1 1-e 0+e 0+e],[0 1 1 1-e 1-e 0+e],c3);plot([0 1 1 0 0],[0 0 1 1 0]);
  wires:
  "p{1}"/1 -> Delay 1/1
  Delay 1/1 -> mux/1
  mux/1 -> "pd{1,1}"/1

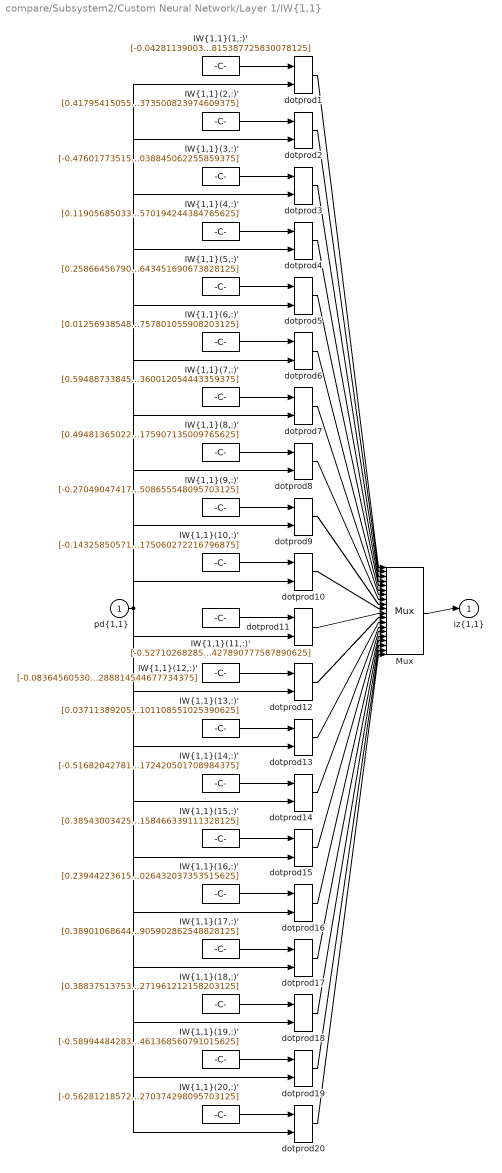
== system compare/Subsystem2/Custom Neural Network/Layer 1/IW{1,1} ==
  "pd{1,1}" : Inport  PortDimensions=4  SampleTime=1
      mask Display: e = 0.06;c1 = [120 230 180]/255;c2 = ([120 230 180]+0)/(256+128);c3 = ([120 230 180]+128)/(256+128);patch([0 1 1 0],[0 0 1 1],c1);patch([0 1 1 1-e 1-e 0+e],[0 0 1 1-e 0+e 0+e],c2);patch([0 0 1 1-e 0+e 0+e],[0 1 1 1-e 1-e 0+e],c3);plot([0 1 1 0 0],[0 0 1 1 0]);
  "IW{1,1}(1,:)'" : Constant  Value=[-0.042811390033023755119501174704055301845073699951171875;-0.34494124940580495053410459149745292961597442626953125;0.212181792987700124086813957546837627887725830078125;0.19703731840338456482442097694729454815387725830078125]
      mask Display: e = 0.06;c1 = [120 150 230]/255;c2 = ([120 150 230]+0)/383;c3 = ([120 150 230]+128)/383;patch([0 1 1 0],[0 0 1 1],c1);patch([0 1 1 1-e 1-e 0+e],[0 0 1 1-e 0+e 0+e],c2);patch([0 0 1 1-e 0+e 0+e],[0 1 1 1-e 1-e 0+e],c3);plot([0 1 1 0 0],[0 0 1 1 0]);disp('Weights');
  "IW{1,1}(10,:)'" : Constant  Value=[-0.1432585057147908458308194212804664857685565948486328125;-0.153266205858384185756193573979544453322887420654296875;0.49559029394590659034491864076699130237102508544921875;-0.07933482509106119795472267242075758986175060272216796875]
      mask Display: e = 0.06;c1 = [120 150 230]/255;c2 = ([120 150 230]+0)/383;c3 = ([120 150 230]+128)/383;patch([0 1 1 0],[0 0 1 1],c1);patch([0 1 1 1-e 1-e 0+e],[0 0 1 1-e 0+e 0+e],c2);patch([0 0 1 1-e 0+e 0+e],[0 1 1 1-e 1-e 0+e],c3);plot([0 1 1 0 0],[0 0 1 1 0]);disp('Weights');
  "IW{1,1}(11,:)'" : Constant  Value=[-0.5271026828588116774909622108680196106433868408203125;-0.19376380367271484050917251806822605431079864501953125;-0.50126266277864350850990149410790763795375823974609375;-0.1275131171211906500051469492973410524427890777587890625]
      mask Display: e = 0.06;c1 = [120 150 230]/255;c2 = ([120 150 230]+0)/383;c3 = ([120 150 230]+128)/383;patch([0 1 1 0],[0 0 1 1],c1);patch([0 1 1 1-e 1-e 0+e],[0 0 1 1-e 0+e 0+e],c2);patch([0 0 1 1-e 0+e 0+e],[0 1 1 1-e 1-e 0+e],c3);plot([0 1 1 0 0],[0 0 1 1 0]);disp('Weights');
  "IW{1,1}(12,:)'" : Constant  Value=[-0.083645605300920744529236117159598506987094879150390625;0.1272107414484172360769065335261984728276729583740234375;-0.1374343203091800968973501539949211291968822479248046875;0.66581955393483605032400873824371956288814544677734375]
      mask Display: e = 0.06;c1 = [120 150 230]/255;c2 = ([120 150 230]+0)/383;c3 = ([120 150 230]+128)/383;patch([0 1 1 0],[0 0 1 1],c1);patch([0 1 1 1-e 1-e 0+e],[0 0 1 1-e 0+e 0+e],c2);patch([0 0 1 1-e 0+e 0+e],[0 1 1 1-e 1-e 0+e],c3);plot([0 1 1 0 0],[0 0 1 1 0]);disp('Weights');
  "IW{1,1}(13,:)'" : Constant  Value=[0.03711389205480629394084957084487541578710079193115234375;-0.462899083442104508634429294033907353878021240234375;-0.2264716472284484527488501726111280731856822967529296875;0.4688615702267180385121037033968605101108551025390625]
      mask Display: e = 0.06;c1 = [120 150 230]/255;c2 = ([120 150 230]+0)/383;c3 = ([120 150 230]+128)/383;patch([0 1 1 0],[0 0 1 1],c1);patch([0 1 1 1-e 1-e 0+e],[0 0 1 1-e 0+e 0+e],c2);patch([0 0 1 1-e 0+e 0+e],[0 1 1 1-e 1-e 0+e],c3);plot([0 1 1 0 0],[0 0 1 1 0]);disp('Weights');
  "IW{1,1}(14,:)'" : Constant  Value=[-0.5168204278140742236047344704275019466876983642578125;0.45663111946031242904808777893777005374431610107421875;-0.51419835913847655728403651664848439395427703857421875;-0.09691171847871636602089751022504060529172420501708984375]
      mask Display: e = 0.06;c1 = [120 150 230]/255;c2 = ([120 150 230]+0)/383;c3 = ([120 150 230]+128)/383;patch([0 1 1 0],[0 0 1 1],c1);patch([0 1 1 1-e 1-e 0+e],[0 0 1 1-e 0+e 0+e],c2);patch([0 0 1 1-e 0+e 0+e],[0 1 1 1-e 1-e 0+e],c3);plot([0 1 1 0 0],[0 0 1 1 0]);disp('Weights');
  "IW{1,1}(15,:)'" : Constant  Value=[0.385430034255971387668893157751881517469882965087890625;-0.215305325209396214436452510199160315096378326416015625;-0.1868848258074100876502399160017375834286212921142578125;0.39665474045523041457528279352118261158466339111328125]
      mask Display: e = 0.06;c1 = [120 150 230]/255;c2 = ([120 150 230]+0)/383;c3 = ([120 150 230]+128)/383;patch([0 1 1 0],[0 0 1 1],c1);patch([0 1 1 1-e 1-e 0+e],[0 0 1 1-e 0+e 0+e],c2);patch([0 0 1 1-e 0+e 0+e],[0 1 1 1-e 1-e 0+e],c3);plot([0 1 1 0 0],[0 0 1 1 0]);disp('Weights');
  "IW{1,1}(16,:)'" : Constant  Value=[0.2394422361532615173285165610650437884032726287841796875;0.5573707637317522056719099055044353008270263671875;-0.44328627858535185612964824031223542988300323486328125;-0.20052230029704232183718204396427609026432037353515625]
      mask Display: e = 0.06;c1 = [120 150 230]/255;c2 = ([120 150 230]+0)/383;c3 = ([120 150 230]+128)/383;patch([0 1 1 0],[0 0 1 1],c1);patch([0 1 1 1-e 1-e 0+e],[0 0 1 1-e 0+e 0+e],c2);patch([0 0 1 1-e 0+e 0+e],[0 1 1 1-e 1-e 0+e],c3);plot([0 1 1 0 0],[0 0 1 1 0]);disp('Weights');
  "IW{1,1}(17,:)'" : Constant  Value=[0.38901068644869807311437170938006602227687835693359375;-0.427525166182410376602973656190442852675914764404296875;-0.443132878250084905058514550546533428132534027099609375;0.37252488448668785725459429158945567905902862548828125]
      mask Display: e = 0.06;c1 = [120 150 230]/255;c2 = ([120 150 230]+0)/383;c3 = ([120 150 230]+128)/383;patch([0 1 1 0],[0 0 1 1],c1);patch([0 1 1 1-e 1-e 0+e],[0 0 1 1-e 0+e 0+e],c2);patch([0 0 1 1-e 0+e 0+e],[0 1 1 1-e 1-e 0+e],c3);plot([0 1 1 0 0],[0 0 1 1 0]);disp('Weights');
  "IW{1,1}(18,:)'" : Constant  Value=[0.38837513753777053171489797023241408169269561767578125;-0.329414929396628364255406040683737955987453460693359375;0.447224063257221360334625614996184594929218292236328125;-0.293902664542561364857675698658567853271961212158203125]
      mask Display: e = 0.06;c1 = [120 150 230]/255;c2 = ([120 150 230]+0)/383;c3 = ([120 150 230]+128)/383;patch([0 1 1 0],[0 0 1 1],c1);patch([0 1 1 1-e 1-e 0+e],[0 0 1 1-e 0+e 0+e],c2);patch([0 0 1 1-e 0+e 0+e],[0 1 1 1-e 1-e 0+e],c3);plot([0 1 1 0 0],[0 0 1 1 0]);disp('Weights');
  "IW{1,1}(19,:)'" : Constant  Value=[-0.58994484283590320483625646375003270804882049560546875;-0.4543619457979339859576839444343931972980499267578125;-0.38699246687251276366481533841579221189022064208984375;-0.1299714765164118601692422316773445345461368560791015625]
      mask Display: e = 0.06;c1 = [120 150 230]/255;c2 = ([120 150 230]+0)/383;c3 = ([120 150 230]+128)/383;patch([0 1 1 0],[0 0 1 1],c1);patch([0 1 1 1-e 1-e 0+e],[0 0 1 1-e 0+e 0+e],c2);patch([0 0 1 1-e 0+e 0+e],[0 1 1 1-e 1-e 0+e],c3);plot([0 1 1 0 0],[0 0 1 1 0]);disp('Weights');
  "IW{1,1}(2,:)'" : Constant  Value=[0.417954150552907910398658941630856133997440338134765625;0.37950717584964566153615805887966416776180267333984375;-0.444355699691141747820211094222031533718109130859375;0.40455774770315766630801590508781373500823974609375]
      mask Display: e = 0.06;c1 = [120 150 230]/255;c2 = ([120 150 230]+0)/383;c3 = ([120 150 230]+128)/383;patch([0 1 1 0],[0 0 1 1],c1);patch([0 1 1 1-e 1-e 0+e],[0 0 1 1-e 0+e 0+e],c2);patch([0 0 1 1-e 0+e 0+e],[0 1 1 1-e 1-e 0+e],c3);plot([0 1 1 0 0],[0 0 1 1 0]);disp('Weights');
  "IW{1,1}(20,:)'" : Constant  Value=[-0.56281218572056845861339979819604195654392242431640625;-0.1531865678348197923330786807127879001200199127197265625;0.32894636374948527102191064841463230550289154052734375;-0.11506127596662703294061458336727810092270374298095703125]
      mask Display: e = 0.06;c1 = [120 150 230]/255;c2 = ([120 150 230]+0)/383;c3 = ([120 150 230]+128)/383;patch([0 1 1 0],[0 0 1 1],c1);patch([0 1 1 1-e 1-e 0+e],[0 0 1 1-e 0+e 0+e],c2);patch([0 0 1 1-e 0+e 0+e],[0 1 1 1-e 1-e 0+e],c3);plot([0 1 1 0 0],[0 0 1 1 0]);disp('Weights');
  "IW{1,1}(3,:)'" : Constant  Value=[-0.476017735150680909583797983941622078418731689453125;0.372659870345571853089694513982976786792278289794921875;0.15761264234491967339835127859259955585002899169921875;-0.301498932852593437559107769629918038845062255859375]
      mask Display: e = 0.06;c1 = [120 150 230]/255;c2 = ([120 150 230]+0)/383;c3 = ([120 150 230]+128)/383;patch([0 1 1 0],[0 0 1 1],c1);patch([0 1 1 1-e 1-e 0+e],[0 0 1 1-e 0+e 0+e],c2);patch([0 0 1 1-e 0+e 0+e],[0 1 1 1-e 1-e 0+e],c3);plot([0 1 1 0 0],[0 0 1 1 0]);disp('Weights');
  "IW{1,1}(4,:)'" : Constant  Value=[0.1190568503323596039056297968272701837122440338134765625;0.025251810519317963166230356364394538104534149169921875;-0.01463313633015732827258315040808156481944024562835693359375;0.0799177967721290960501079325695172883570194244384765625]
      mask Display: e = 0.06;c1 = [120 150 230]/255;c2 = ([120 150 230]+0)/383;c3 = ([120 150 230]+128)/383;patch([0 1 1 0],[0 0 1 1],c1);patch([0 1 1 1-e 1-e 0+e],[0 0 1 1-e 0+e 0+e],c2);patch([0 0 1 1-e 0+e 0+e],[0 1 1 1-e 1-e 0+e],c3);plot([0 1 1 0 0],[0 0 1 1 0]);disp('Weights');
  "IW{1,1}(5,:)'" : Constant  Value=[0.2586645679057075764006867757416330277919769287109375;-0.359798037926290892318803571470198221504688262939453125;0.49791321437721602904957762802951037883758544921875;-0.2408924072199911947667061440370162017643451690673828125]
      mask Display: e = 0.06;c1 = [120 150 230]/255;c2 = ([120 150 230]+0)/383;c3 = ([120 150 230]+128)/383;patch([0 1 1 0],[0 0 1 1],c1);patch([0 1 1 1-e 1-e 0+e],[0 0 1 1-e 0+e 0+e],c2);patch([0 0 1 1-e 0+e 0+e],[0 1 1 1-e 1-e 0+e],c3);plot([0 1 1 0 0],[0 0 1 1 0]);disp('Weights');
  "IW{1,1}(6,:)'" : Constant  Value=[0.01256938548635226811367449073486568522639572620391845703125;0.422855987628569407466017082697362639009952545166015625;0.482605939133784911376778836711309850215911865234375;-0.478909325852367839804202276354772038757801055908203125]
      mask Display: e = 0.06;c1 = [120 150 230]/255;c2 = ([120 150 230]+0)/383;c3 = ([120 150 230]+128)/383;patch([0 1 1 0],[0 0 1 1],c1);patch([0 1 1 1-e 1-e 0+e],[0 0 1 1-e 0+e 0+e],c2);patch([0 0 1 1-e 0+e 0+e],[0 1 1 1-e 1-e 0+e],c3);plot([0 1 1 0 0],[0 0 1 1 0]);disp('Weights');
  "IW{1,1}(7,:)'" : Constant  Value=[0.5948873384524977492304742554551921784877777099609375;0.281306962804711513381761278651538304984569549560546875;-0.1572109737119190830956227955539361573755741119384765625;0.1660798915358044636203516120076528750360012054443359375]
      mask Display: e = 0.06;c1 = [120 150 230]/255;c2 = ([120 150 230]+0)/383;c3 = ([120 150 230]+128)/383;patch([0 1 1 0],[0 0 1 1],c1);patch([0 1 1 1-e 1-e 0+e],[0 0 1 1-e 0+e 0+e],c2);patch([0 0 1 1-e 0+e 0+e],[0 1 1 1-e 1-e 0+e],c3);plot([0 1 1 0 0],[0 0 1 1 0]);disp('Weights');
  "IW{1,1}(8,:)'" : Constant  Value=[0.494813650227310108942191391179221682250499725341796875;-0.1661270735577930202087060251869843341410160064697265625;-0.323120860559985623172707391859148629009723663330078125;-0.120857806854206606406165747102932073175907135009765625]
      mask Display: e = 0.06;c1 = [120 150 230]/255;c2 = ([120 150 230]+0)/383;c3 = ([120 150 230]+128)/383;patch([0 1 1 0],[0 0 1 1],c1);patch([0 1 1 1-e 1-e 0+e],[0 0 1 1-e 0+e 0+e],c2);patch([0 0 1 1-e 0+e 0+e],[0 1 1 1-e 1-e 0+e],c3);plot([0 1 1 0 0],[0 0 1 1 0]);disp('Weights');
  "IW{1,1}(9,:)'" : Constant  Value=[-0.27049047417204652443700751973665319383144378662109375;-0.030493674231205934732624740490791737101972103118896484375;-0.30275890613240985516085856943391263484954833984375;0.32392632672577914565437140481662936508655548095703125]
      mask Display: e = 0.06;c1 = [120 150 230]/255;c2 = ([120 150 230]+0)/383;c3 = ([120 150 230]+128)/383;patch([0 1 1 0],[0 0 1 1],c1);patch([0 1 1 1-e 1-e 0+e],[0 0 1 1-e 0+e 0+e],c2);patch([0 0 1 1-e 0+e 0+e],[0 1 1 1-e 1-e 0+e],c3);plot([0 1 1 0 0],[0 0 1 1 0]);disp('Weights');
  Mux : Mux  Inputs=20
      mask Display: e = 0.06;c1 = [120 150 230]/255;c2 = ([120 150 230]+0)/383;c3 = ([120 150 230]+128)/383;patch([0 1 1 0],[0 0 1 1],c1);patch([0 1 1 1-e 1-e 0+e],[0 0 1 1-e 0+e 0+e],c2);patch([0 0 1 1-e 0+e 0+e],[0 1 1 1-e 1-e 0+e],c3);plot([0 1 1 0 0],[0 0 1 1 0]);disp('Mux');
  dotprod{1..20} (20 alike) : neural/Weight Functions/dotprod
  "iz{1,1}" : Outport
      mask Display: e = 0.06;c1 = [120 230 180]/255;c2 = ([120 230 180]+0)/(256+128);c3 = ([120 230 180]+128)/(256+128);patch([0 1 1 0],[0 0 1 1],c1);patch([0 1 1 1-e 1-e 0+e],[0 0 1 1-e 0+e 0+e],c2);patch([0 0 1 1-e 0+e 0+e],[0 1 1 1-e 1-e 0+e],c3);plot([0 1 1 0 0],[0 0 1 1 0]);
  wires:
  "IW{1,1}(1,:)'"/1 -> dotprod1/1
  "pd{1,1}"/1 -> dotprod1/2, dotprod2/2, dotprod3/2, dotprod4/2, dotprod5/2, dotprod6/2, dotprod7/2, dotprod8/2, dotprod9/2, dotprod10/2, dotprod11/2, dotprod12/2, dotprod13/2, dotprod14/2, dotprod15/2, dotprod16/2, dotprod17/2, dotprod18/2, dotprod19/2, dotprod20/2
  dotprod1/1 -> Mux/1
  "IW{1,1}(2,:)'"/1 -> dotprod2/1
  dotprod2/1 -> Mux/2
  "IW{1,1}(3,:)'"/1 -> dotprod3/1
  dotprod3/1 -> Mux/3
  "IW{1,1}(4,:)'"/1 -> dotprod4/1
  dotprod4/1 -> Mux/4
  "IW{1,1}(5,:)'"/1 -> dotprod5/1
  dotprod5/1 -> Mux/5
  "IW{1,1}(6,:)'"/1 -> dotprod6/1
  dotprod6/1 -> Mux/6
  "IW{1,1}(7,:)'"/1 -> dotprod7/1
  dotprod7/1 -> Mux/7
  "IW{1,1}(8,:)'"/1 -> dotprod8/1
  dotprod8/1 -> Mux/8
  "IW{1,1}(9,:)'"/1 -> dotprod9/1
  dotprod9/1 -> Mux/9
  "IW{1,1}(10,:)'"/1 -> dotprod10/1
  dotprod10/1 -> Mux/10
  "IW{1,1}(11,:)'"/1 -> dotprod11/1
  dotprod11/1 -> Mux/11
  "IW{1,1}(12,:)'"/1 -> dotprod12/1
  dotprod12/1 -> Mux/12
  "IW{1,1}(13,:)'"/1 -> dotprod13/1
  dotprod13/1 -> Mux/13
  "IW{1,1}(14,:)'"/1 -> dotprod14/1
  dotprod14/1 -> Mux/14
  "IW{1,1}(15,:)'"/1 -> dotprod15/1
  dotprod15/1 -> Mux/15
  "IW{1,1}(16,:)'"/1 -> dotprod16/1
  dotprod16/1 -> Mux/16
  "IW{1,1}(17,:)'"/1 -> dotprod17/1
  dotprod17/1 -> Mux/17
  "IW{1,1}(18,:)'"/1 -> dotprod18/1
  dotprod18/1 -> Mux/18
  "IW{1,1}(19,:)'"/1 -> dotprod19/1
  dotprod19/1 -> Mux/19
  "IW{1,1}(20,:)'"/1 -> dotprod20/1
  dotprod20/1 -> Mux/20
  Mux/1 -> "iz{1,1}"/1
